simulink model "QCar2_CameraDriving"  (R2025b)
settings: Solver=ode2  StartTime=0.0  StopTime=inf  FixedStep=1/100  RelTol=1e-3  EnableMultiTasking=on
InitFcn:
  | modelFile = get_param(bdroot,'FileName');
  | modelDir  = fileparts(modelFile);
  | 
  | addpath(modelDir); % so load_waypoints.m is found if it sits next to the model
  | addpath(fullfile(modelDir,".."));
  | 
  | wpFile = fullfile(modelDir, "waypoints.txt");
  | WP = load_waypoints(wpFile);
  | 
  | assignin("base","WP",WP);
model workspace (MAT data in the model file):
  camera_rate : Simulink.Parameter (value not decoded)
  depth_rate : Simulink.Parameter (value not decoded)
symbols that are objects in the model workspace (value not decoded): camera_rate, depth_rate
undefined symbols (not defined in the file or in its folder): gcbh, HIL, JPEG, Point, qc_get_step_size, Video3D, video_display_show
libraries: quarc_library x37, simulink x14
(part 2 of 3)

== system QCar2_CameraDriving/monitorTiming 2 ==
  note: moniorTiming Module:
      |
      | This subsystem outputs the sample time and computation time of the model.
      |
      | Outputs:
      | sampleTime (s) n/a : Sample time (unfiltered and filtered) in seconds.
      | computationTime (s) n/a : Computation time (unfiltered and filtered) in seconds.
      |
      | Usage:
      | Compare the Sample Time (s) output to a constant (qc_get_step_size) to monitor whether or not the desired sample time is being achieved. The Computation Time (s) values should be lower than the corresponding sample time value to ensure that the solver has enough time per time step.
  note: Timing Performance
  Computation Time : quarc_library/Sources/Time/Computation Time  sample_time=depth_rate  use_model=on  use_cpu_time=off
  Constant : Constant  Value=depth_rate  SampleTime=depth_rate
  Mux : Mux  Inputs=2
  Sample Time : quarc_library/Sources/Time/Sample Time  Priority=-99  sample_time=depth_rate
  sampleTime (s) : Outport  VectorParamsAs1DForOutWhenUnconnected=off
  computationTime (s) : Outport  Port=2  VectorParamsAs1DForOutWhenUnconnected=off
  wires:
  Constant/1 -> Mux/2
  Sample Time/1 -> Mux/1
  Mux/1 -> sampleTime (s)/1
  Computation Time/1 -> computationTime (s)/1

== system QCar2_CameraDriving/monitorTiming 3 ==
  note: Timing Performance
  note: monitorTiming Module:
      |
      | This subsystem provides three timing signals for any given rate in your model.
      |
      | Outputs:
      | timing (s) n/a : Sample time, sample time reference and computation time in seconds.
      |
      | Usage:
      | Set the 'Sample time (seconds)' parameter in all three blocks below to the same number. This will provide the actual sample time at each time step, the reference sample time that is being targeted as well as the computation time of that particular loop in the model into one vector signal for scoping.
  Computation Time : quarc_library/Sources/Time/Computation Time  sample_time=qc_get_step_size  use_model=on  use_cpu_time=off
  Constant : Constant  Value=qc_get_step_size
  Mux : Mux  Inputs=3
  Sample Time : quarc_library/Sources/Time/Sample Time  Priority=-99  sample_time=qc_get_step_size
  timing (s) : Outport  VectorParamsAs1DForOutWhenUnconnected=off
  wires:
  Mux/1 -> timing (s)/1
  Computation Time/1 -> Mux/3  "computation time"
  Sample Time/1 -> Mux/1  "actual sample time"
  Constant/1 -> Mux/2  "reference"

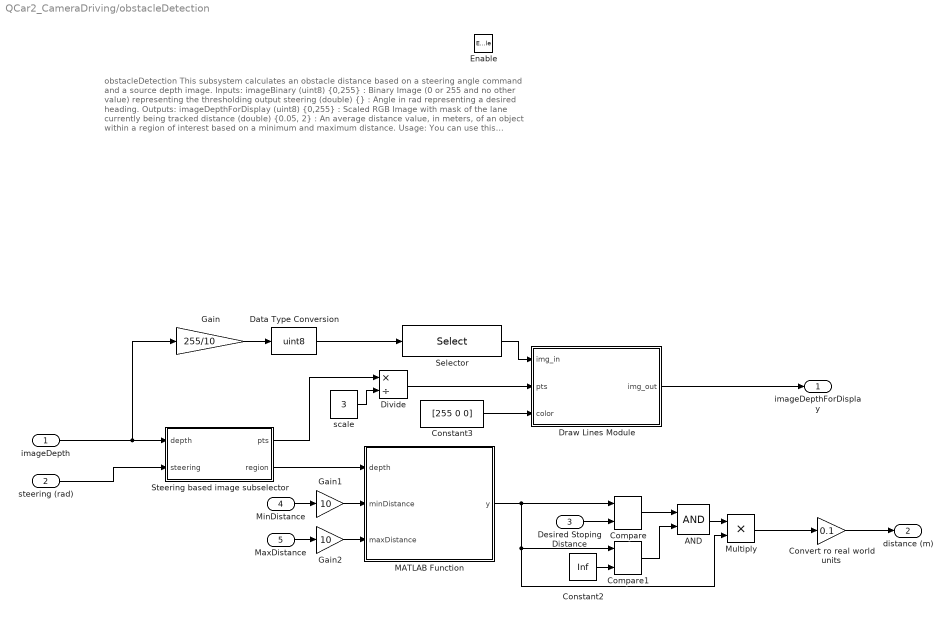
== system QCar2_CameraDriving/obstacleDetection ==
  note: obstacleDetection
      | This subsystem calculates an obstacle distance based on a steering angle command and a source depth image.
      |
      | Inputs:
      | imageBinary (uint8) {0,255} : Binary Image (0 or 255 and no other value) representing the thresholding output
      | steering (double) {} : Angle in rad representing a desired heading.
      |
      | Outputs:
      | imageDepthForDisplay (uint8) {0,255} : Scaled RGB Image with mask of the lane currently being tracked
      | distance (double) {0.05, 2} : An average distance value, in meters, of an object within a region of interest based on a minimum and maximum distance.
      |
      | Usage:
      |
      | You can use this subsystem to determine if the desired heading angle will cause the car to colllide with an obstacle by examining the distances from a region of interest within the depth image and calculating how far the obstacle is.
  imageDepth : Inport
  steering (rad) : Inport  Port=2
  Desired Stoping Distance : Inport  Port=3
  MinDistance : Inport  Port=4
  MaxDistance : Inport  Port=5
  Enable : EnablePort  PropagateVarSize=During execution
  AND : Logic  AllPortsSameDT=off  OutDataTypeStr=boolean
  Compare : quarc_library/Logic Operations/Compare  operator=>=  output_data_type=boolean
      settings: SourceProductName=QUARC Targets
  Compare1 : quarc_library/Logic Operations/Compare  operator=<  output_data_type=boolean
      settings: SourceProductName=QUARC Targets
  Constant2 : Constant  Value=Inf
  Constant3 : Constant  Value=[255 0 0]
  Convert ro real world units : Gain  Gain=0.1
  Data Type Conversion : DataTypeConversion  OutDataTypeStr=uint8  SaturateOnIntegerOverflow=off  RndMeth=Floor
  Divide : Product  Inputs=*/  OutDataTypeStr=Inherit: Inherit via back propagation
  Draw Lines Module : MATLAB Function  TreatAsAtomicUnit=on
  Gain : Gain  Gain=255/10
  Gain1 : Gain  Gain=10
  Gain2 : Gain  Gain=10
  MATLAB Function : MATLAB Function  TreatAsAtomicUnit=on
  Multiply : Product
  Selector : Selector  NumberOfDimensions=2  InputPortWidth=3  IndexOptions=Index vector (dialog),Index vector (dialog)  Indices=[1:3:360],[1:3:640]  OutputSizes=1,1
  Steering based image subselector : MATLAB Function  TreatAsAtomicUnit=on
  scale : Constant  Value=3
  imageDepthForDisplay : Outport  VectorParamsAs1DForOutWhenUnconnected=off
  distance (m) : Outport  Port=2  VectorParamsAs1DForOutWhenUnconnected=off
  wires:
  Constant3/1 -> Draw Lines Module/3(color)
  Steering based image subselector/1(pts) -> Divide/1
  Steering based image subselector/2(region) -> MATLAB Function/1(depth)
  steering (rad)/1 -> Steering based image subselector/2(steering)
  Multiply/1 -> Convert ro real world units/1
  MaxDistance/1 -> Gain2/1
  MinDistance/1 -> Gain1/1
  MATLAB Function/1(y) -> Compare/1, Multiply/2, Compare1/1
  imageDepth/1 -> Steering based image subselector/1(depth), Gain/1
  Selector/1 -> Draw Lines Module/1(img_in)
  Data Type Conversion/1 -> Selector/1
  Divide/1 -> Draw Lines Module/2(pts)
  Draw Lines Module/1(img_out) -> imageDepthForDisplay/1
  scale/1 -> Divide/2
  Gain/1 -> Data Type Conversion/1
  Desired Stoping Distance/1 -> Compare/2
  Compare/1 -> AND/1
  Compare1/1 -> AND/2
  Constant2/1 -> Compare1/2
  AND/1 -> Multiply/1
  Convert ro real world units/1 -> distance (m)/1
  Gain1/1 -> MATLAB Function/2(minDistance)
  Gain2/1 -> MATLAB Function/3(maxDistance)

== system QCar2_CameraDriving/odometry ==
  v_in : Inport
  steer_in : Inport  Port=2
  Ts_const : Constant  Value=0.02
  odometry_step : MATLAB Function  TreatAsAtomicUnit=on
  state_delay : UnitDelay  InitialCondition=[0;0;0]  SampleTime=-1  HasFrameUpgradeWarning=on
  pose_out : Outport
  wires:
  state_delay/1 -> odometry_step/1(prev_state)
  v_in/1 -> odometry_step/2(v)
  steer_in/1 -> odometry_step/3(steer)
  Ts_const/1 -> odometry_step/4(Ts)
  odometry_step/1(pose_next) -> state_delay/1, pose_out/1

== system QCar2_CameraDriving/pointCloud ==
  note: Convert LIDAR information to Point Cloud Image
  note: pointCloud Module:
      |
      | This subsystem generates a point cloud image based on LIDAR data.
      |
      | Inputs:
      | distances (m) n/a : Distances measured by LIDAR
      | headings (rad) n/a : Headings at which distances are measured
      |
      | Outputs:
      | map (px) {0, 1} : 400 x 400 point cloud image
      |
      | Usage:
      | The data is dynamically saturated based on the maximumDistance (m) constant. To prevent a circle with radius being the maximumDistance showing up in the point cloud as a result of this saturation, data points corresponding to this are dropped in the findXYContour function. The function contourToPointCloud updates pixels in the map to 1 at new locations, and decays older data at the rate specified by the decay parameter.
  distances (m) : Inport
  heading (rad) : Inport  Port=2
  Constant1 : Constant  Value=0
  Saturation Dynamic : simulink/Discontinuities/Saturation Dynamic  OutMin=[]  OutMax=[]  OutDataTypeStr=Inherit: Same as second input  OutDataType=fixdt(1, 16)  OutScaling=2^-10  DoSatur=off
  contourToPointCloud : MATLAB Function  TreatAsAtomicUnit=on
  decay : Constant  Value=0
  findXYContour : MATLAB Function  TreatAsAtomicUnit=on
  maximumDistance (m) : Constant  Value=4
  map : Outport  VectorParamsAs1DForOutWhenUnconnected=off
  wires:
  distances (m)/1 -> Saturation Dynamic/2
  contourToPointCloud/1(mapOut) -> map/1
  Saturation Dynamic/1 -> findXYContour/1(distances)
  maximumDistance (m)/1 -> findXYContour/3(d_max), Saturation Dynamic/1
  Constant1/1 -> Saturation Dynamic/3
  decay/1 -> contourToPointCloud/3(decay)
  findXYContour/1(X) -> contourToPointCloud/1(X)
  findXYContour/2(Y) -> contourToPointCloud/2(Y)
  heading (rad)/1 -> findXYContour/2(heading)

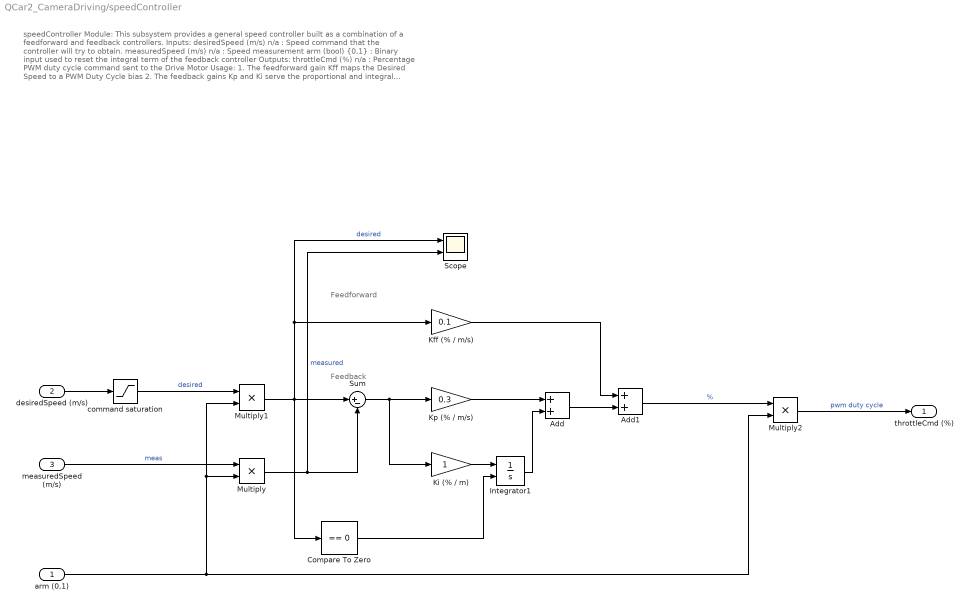
== system QCar2_CameraDriving/speedController ==
  note: Feedforward
  note: Feedback
  note: speedController Module:
      |
      | This subsystem provides a general speed controller built as a combination of a feedforward and feedback controllers.
      |
      | Inputs:
      | desiredSpeed (m/s) n/a : Speed command that the controller will try to obtain.
      | measuredSpeed (m/s) n/a : Speed measurement
      | arm (bool) {0,1} : Binary input used to reset the integral term of the feedback controller
      |
      | Outputs:
      | throttleCmd (%) n/a : Percentage PWM duty cycle command sent to the Drive Motor
      |
      | Usage:
      | 1. The feedforward gain Kff maps the Desired Speed to a PWM Duty Cycle bias
      | 2. The feedback gains Kp and Ki serve the proportional and integral terms to output corrections to the PWM Duty Cycle so as to regulate the desired speed.
  arm (0,1) : Inport
  desiredSpeed (m/s) : Inport  Port=2
  measuredSpeed (m/s) : Inport  Port=3
  Add : Sum
  Add1 : Sum
  Compare To Zero : simulink/Logic and Bit Operations/Compare To Zero  relop===  OutDataTypeStr=boolean
  Integrator1 : Integrator  ExternalReset=either  LimitOutput=on  UpperSaturationLimit=0.4  LowerSaturationLimit=-0.4
  Kff (% / m/s) : Gain  Gain=0.1
  "Ki (% / m) " : Gain
  Kp (% / m/s) : Gain  Gain=0.3
  Multiply : Product
  Multiply1 : Product
  Multiply2 : Product
  Scope : Scope  NumInputPorts=2
      settings: Title=Control Performance  ActiveDisplayYMinimum=0.76298814046961727  ActiveDisplayYMaximum=2.5122465814768962  YLabel=m/s
  Sum : Sum  Inputs=|+-
  command saturation : Saturate  UpperLimit=5  LowerLimit=-5
  throttleCmd (%) : Outport  VectorParamsAs1DForOutWhenUnconnected=off
  wires:
  command saturation/1 -> Multiply1/1  "desired"
  arm (0,1)/1 -> Multiply1/2, Multiply/2, Multiply2/2
  measuredSpeed (m/s)/1 -> Multiply/1  "meas"
  Multiply/1 -> Sum/2, Scope/2  "measured"
  Add/1 -> Add1/2
  Add1/1 -> Multiply2/1  "%"
  Multiply1/1 -> Compare To Zero/1, Sum/1, Kff (% / m/s)/1, Scope/1  "desired"
  Integrator1/1 -> Add/2
  Multiply2/1 -> throttleCmd (%)/1  "pwm duty cycle"
  Kp (% / m/s)/1 -> Add/1
  Compare To Zero/1 -> Integrator1/2
  Kff (% / m/s)/1 -> Add1/1
  Sum/1 -> "Ki (% / m) "/1, Kp (% / m/s)/1
  "Ki (% / m) "/1 -> Integrator1/1
  desiredSpeed (m/s)/1 -> command saturation/1

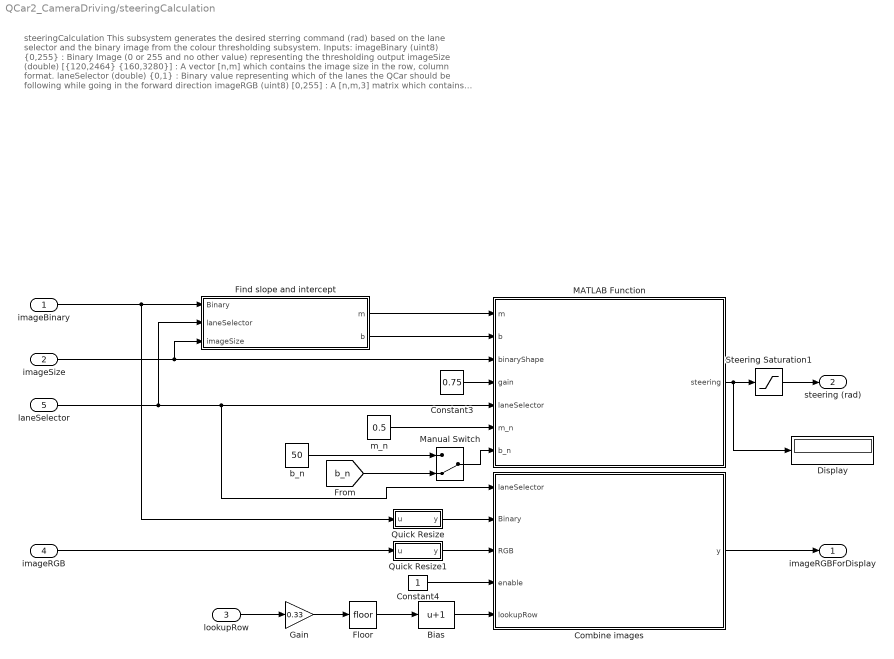
== system QCar2_CameraDriving/steeringCalculation ==
  note: steeringCalculation
      | This subsystem generates the desired sterring command (rad) based on the lane selector and the binary image from the colour thresholding subsystem.
      |
      | Inputs:
      | imageBinary (uint8) {0,255} : Binary Image (0 or 255 and no other value) representing the thresholding output
      | imageSize (double) [{120,2464} {160,3280}] : A vector [n,m] which contains the image size in the row, column format.
      | laneSelector (double) {0,1} : Binary value representing which of the lanes the QCar should be following while going in the forward direction
      | imageRGB (uint8) [0,255] : A [n,m,3] matrix which contains RGB values of an image in uint8 format
      |
      | Outputs:
      | steering (double) {-0.5,0.5} : Angle in rad representing the desired steering command based on the linearPolyFit
      | imageRGBForDisplay (uint8) {0,255} : A [n,m,3] matrix representing an RGB Image with mask of the lane currently being tracked
      |
      | Usage:
      |
      | This module can be used to generate a desired steering angle based on a thresheld image. A linear polygonal fit is used to generate a slope based on the equation y = mx+b whose slope and y intercept will define the steering angle commanded up to 0.5 (rad). The RGB image is a combination of the binary image holding information of the lane being followed, and a scaled version of the original RGB image.
  imageBinary : Inport
  imageSize : Inport  Port=2
  lookupRow : Inport  Port=3
  imageRGB : Inport  Port=4
  laneSelector : Inport  Port=5
  Bias : Bias  Bias=1  SaturateOnIntegerOverflow=off
  Combine images : MATLAB Function  TreatAsAtomicUnit=on
  Constant3 : Constant  Value=0.75
  Constant4 : Constant
  Display : Display
  Find slope and intercept : MATLAB Function  TreatAsAtomicUnit=on
  Floor : Rounding
  Gain : Gain  Gain=0.33
  MATLAB Function : MATLAB Function  TreatAsAtomicUnit=on
  Manual Switch : ManualSwitch  CurrentSetting=0
  Quick Resize : MATLAB Function  TreatAsAtomicUnit=on
  Quick Resize1 : MATLAB Function  TreatAsAtomicUnit=on
  Steering Saturation1 : Saturate
  b_n : Constant  Value=50
  m_n : Constant  Value=0.5
  imageRGBForDisplay : Outport  VectorParamsAs1DForOutWhenUnconnected=off
  steering (rad) : Outport  Port=2  VectorParamsAs1DForOutWhenUnconnected=off
  wires:
  Find slope and intercept/1(m) -> MATLAB Function/1(m)
  laneSelector/1 -> MATLAB Function/5(laneSelector), Combine images/1(laneSelector), Find slope and intercept/2(laneSelector)
  MATLAB Function/1(steering) -> Display/1, Steering Saturation1/1
  Constant3/1 -> MATLAB Function/4(gain)
  imageBinary/1 -> Quick Resize/1(u), Find slope and intercept/1(Binary)
  Find slope and intercept/2(b) -> MATLAB Function/2(b)
  Constant4/1 -> Combine images/4(enable)
  Quick Resize/1(y) -> Combine images/2(Binary)
  Quick Resize1/1(y) -> Combine images/3(RGB)
  Combine images/1(y) -> imageRGBForDisplay/1
  imageRGB/1 -> Quick Resize1/1(u)
  Steering Saturation1/1 -> steering (rad)/1
  Gain/1 -> Floor/1
  imageSize/1 -> Find slope and intercept/3(imageSize), MATLAB Function/3(binaryShape)
  lookupRow/1 -> Gain/1
  Bias/1 -> Combine images/5(lookupRow)
  Floor/1 -> Bias/1
  b_n/1 -> Manual Switch/1
  Manual Switch/1 -> MATLAB Function/7(b_n)
  [b_n] -> Manual Switch/2
  m_n/1 -> MATLAB Function/6(m_n)

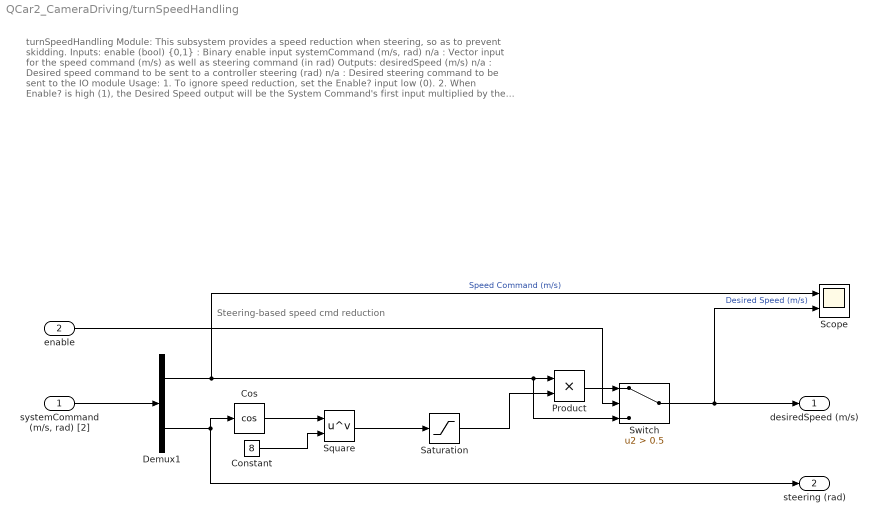
== system QCar2_CameraDriving/turnSpeedHandling ==
  note: turnSpeedHandling Module:
      |
      | This subsystem provides a speed reduction when steering, so as to prevent skidding.
      |
      | Inputs:
      | enable (bool) {0,1} : Binary enable input
      | systemCommand (m/s, rad) n/a : Vector input for the speed command (m/s) as well as steering command (in rad)
      |
      | Outputs:
      | desiredSpeed (m/s) n/a : Desired speed command to be sent to a controller
      | steering (rad) n/a : Desired steering command to be sent to the IO module
      |
      | Usage:
      | 1. To ignore speed reduction, set the Enable? input low (0).
      | 2. When Enable? is high (1), the Desired Speed output will be the System Command's first input multiplied by the cosine of the steering. Note that the lower limit of this reduction is set to 50% of the speed command input.
  note: Steering-based speed cmd reduction
  "systemCommand (m/s, rad) [2]" : Inport
  enable : Inport  Port=2
  Constant : Constant  Value=8
  Cos : Trigonometry  Operator=cos
  Demux1 : Demux  Outputs=2
  Product : Product
  Saturation : Saturate  UpperLimit=1  LowerLimit=0.5
  Scope : Scope  NumInputPorts=2
      settings: Title=Turn-Speed Handling  ActiveDisplayYMinimum=-2  ActiveDisplayYMaximum=2  YLabel=m/s  DataLoggingVariableName=ScopeData2
  Square : Math  Operator=pow  SignedPower=on
  Switch : Switch  Criteria=u2 > Threshold  Threshold=0.5  SaturateOnIntegerOverflow=off  InputSameDT=off
  desiredSpeed (m/s) : Outport  VectorParamsAs1DForOutWhenUnconnected=off
  steering (rad) : Outport  Port=2  VectorParamsAs1DForOutWhenUnconnected=off
  wires:
  Cos/1 -> Square/1
  Switch/1 -> desiredSpeed (m/s)/1, Scope/2  "Desired Speed (m/s)"
  Product/1 -> Switch/1
  Saturation/1 -> Product/2
  Demux1/1 -> Product/1, Switch/3, Scope/1  "Speed Command (m/s)"
  "systemCommand (m/s, rad) [2]"/1 -> Demux1/1
  enable/1 -> Switch/2
  Constant/1 -> Square/2
  Demux1/2 -> steering (rad)/1, Cos/1
  Square/1 -> Saturation/1

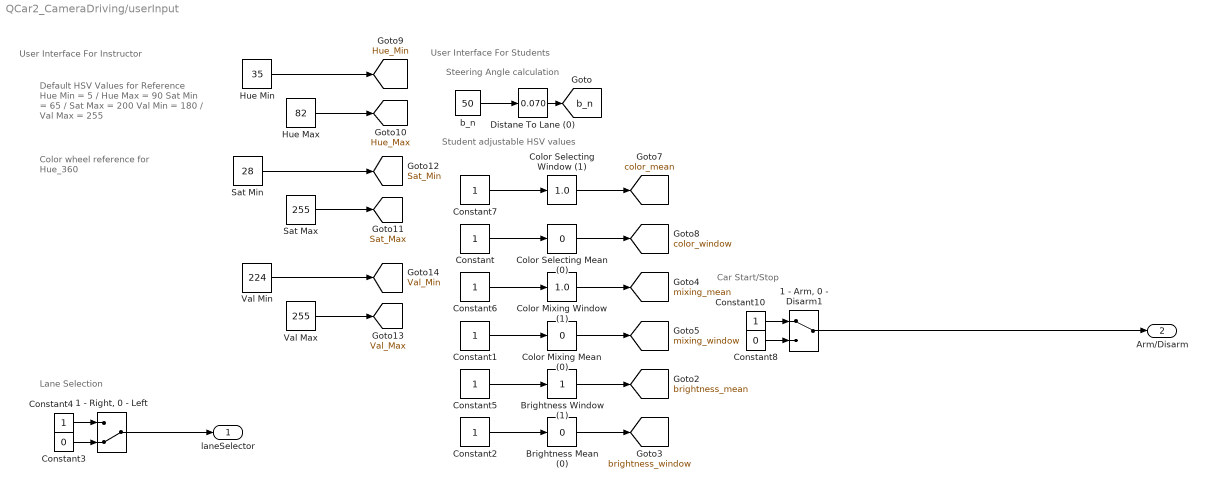
== system QCar2_CameraDriving/userInput ==
  note: Default HSV Values for Reference
      | Hue Min = 5 / Hue Max = 90
      | Sat Min = 65 / Sat Max = 200
      | Val Min = 180 / Val Max = 255
  note: User Interface For Instructor
  note: Student adjustable HSV values
  note: Lane Selection
  note: Car Start/Stop
  note: Steering Angle calculation
  note: User Interface For Students
  note: Color wheel
      | reference
      | for Hue_360
  "1 - Arm, 0 - Disarm1" : ManualSwitch
  "1 - Right, 0 - Left" : ManualSwitch  CurrentSetting=0
  Brightness Mean (0) : simulink/Math Operations/Slider Gain  gain=0  low=-1  high=1
  Brightness Window (1) : simulink/Math Operations/Slider Gain  gain=1  low=0  high=1
  Color Mixing Mean (0) : simulink/Math Operations/Slider Gain  gain=0  low=-1  high=1
  Color Mixing Window (1) : simulink/Math Operations/Slider Gain  gain=1.0  low=0  high=1
  Color Selecting Mean (0) : simulink/Math Operations/Slider Gain  gain=0  low=-1  high=1
  Color Selecting Window (1) : simulink/Math Operations/Slider Gain  gain=1.0  low=0  high=1
  Constant{,1..2,4..7,10} (8 alike) : Constant
  Constant3 : Constant  Value=0
  Constant8 : Constant  Value=0
  "Distane To Lane (0) " : simulink/Math Operations/Slider Gain  gain=0.070  low=0  high=1
  Hue Max : Constant  Value=82
  Hue Min : Constant  Value=35
  Sat Max : Constant  Value=255
  Sat Min : Constant  Value=28
  Val Max : Constant  Value=255
  Val Min : Constant  Value=224
  b_n : Constant  Value=50
  laneSelector : Outport  VectorParamsAs1DForOutWhenUnconnected=off
  Arm/Disarm : Outport  Port=2  VectorParamsAs1DForOutWhenUnconnected=off
  tag scope: Hue_Max=global, Hue_Min=global, Sat_Max=global, Sat_Min=global, Val_Max=global, Val_Min=global, b_n=global, brightness_mean=global, brightness_window=global, color_mean=global, color_window=global, mixing_mean=global, mixing_window=global
  wires:
  Constant3/1 -> "1 - Right, 0 - Left"/2
  "1 - Arm, 0 - Disarm1"/1 -> Arm/Disarm/1
  b_n/1 -> "Distane To Lane (0) "/1
  Constant4/1 -> "1 - Right, 0 - Left"/1
  Constant10/1 -> "1 - Arm, 0 - Disarm1"/1
  "1 - Right, 0 - Left"/1 -> laneSelector/1
  Constant8/1 -> "1 - Arm, 0 - Disarm1"/2
  "Distane To Lane (0) "/1 -> [b_n]
  Color Mixing Window (1)/1 -> [mixing_mean]
  Constant/1 -> Color Selecting Mean (0)/1
  Constant2/1 -> Brightness Mean (0)/1
  Constant5/1 -> Brightness Window (1)/1
  Constant1/1 -> Color Mixing Mean (0)/1
  Color Selecting Mean (0)/1 -> [color_window]
  Brightness Window (1)/1 -> [brightness_mean]
  Color Selecting Window (1)/1 -> [color_mean]
  Brightness Mean (0)/1 -> [brightness_window]
  Color Mixing Mean (0)/1 -> [mixing_window]
  Constant6/1 -> Color Mixing Window (1)/1
  Constant7/1 -> Color Selecting Window (1)/1
  Hue Min/1 -> [Hue_Min]
  Sat Min/1 -> [Sat_Min]
  Val Min/1 -> [Val_Min]
  Hue Max/1 -> [Hue_Max]
  Sat Max/1 -> [Sat_Max]
  Val Max/1 -> [Val_Max]

== system QCar2_CameraDriving/TrafficPerception_Python/TrafficTracking_Filter ==
  tl_state_raw : Inport  OutDataTypeStr=uint8
  stopSign_dist_raw : Inport  Port=2  OutDataTypeStr=double
  stop_required_raw : Inport  Port=3  OutDataTypeStr=boolean
  MATLAB Function : MATLAB Function  TreatAsAtomicUnit=on
  tl_stop : Outport  OutDataTypeStr=boolean
  sign_stop : Outport  Port=2  OutDataTypeStr=boolean
  stopSign_dist : Outport  Port=3  OutDataTypeStr=double
  wires:
  tl_state_raw/1 -> MATLAB Function/1(tl_state_raw)
  stopSign_dist_raw/1 -> MATLAB Function/3(stopSign_dist_raw)
  stop_required_raw/1 -> MATLAB Function/2(stop_required_raw)
  MATLAB Function/1(tl_stop) -> tl_stop/1
  MATLAB Function/2(sign_stop) -> sign_stop/1
  MATLAB Function/3(stopSign_dist) -> stopSign_dist/1

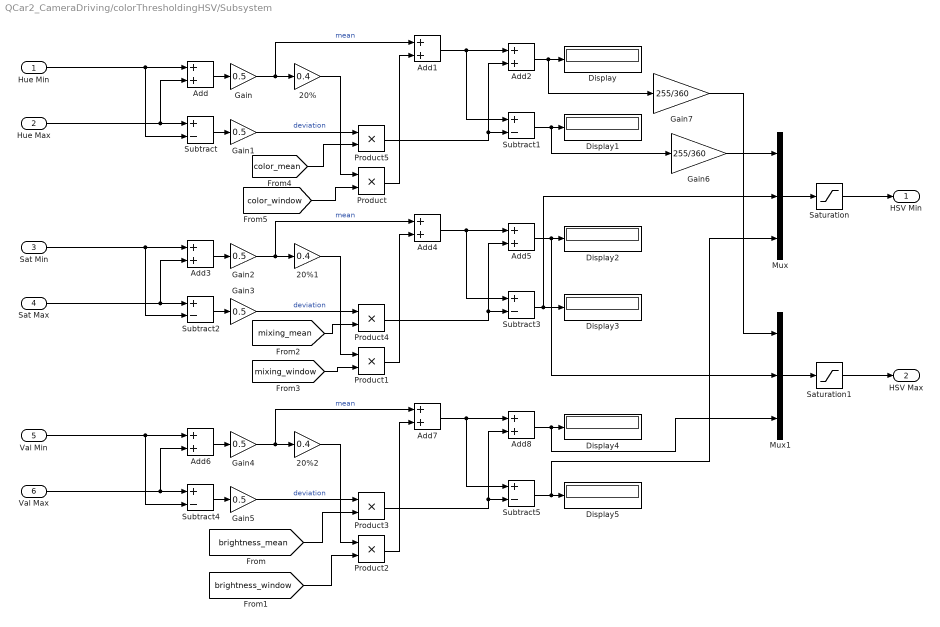
== system QCar2_CameraDriving/colorThresholdingHSV/Subsystem ==
  Hue Min : Inport
  Hue Max : Inport  Port=2
  Sat Min : Inport  Port=3
  Sat Max : Inport  Port=4
  Val Min : Inport  Port=5
  Val Max : Inport  Port=6
  20% : Gain  Gain=0.4
  20%1 : Gain  Gain=0.4
  20%2 : Gain  Gain=0.4
  Add{,1..8} (9 alike) : Sum
  Display{,1..5} (6 alike) : Display
  Gain{,1..5} (6 alike) : Gain  Gain=0.5
  Gain6 : Gain  Gain=255/360
  Gain7 : Gain  Gain=255/360
  Mux : Mux  Inputs=3
  Mux1 : Mux  Inputs=3
  Product{,1..5} (6 alike) : Product
  Saturation : Saturate  UpperLimit=[255 255 255]  LowerLimit=[0 0 0]
  Saturation1 : Saturate  UpperLimit=[255 255 255]  LowerLimit=[0 0 0]
  Subtract{,1..5} (6 alike) : Sum  Inputs=+-
  HSV Min : Outport  VectorParamsAs1DForOutWhenUnconnected=off
  HSV Max : Outport  Port=2  VectorParamsAs1DForOutWhenUnconnected=off
  wires:
  Product1/1 -> Add4/2
  Val Min/1 -> Add6/1, Subtract4/2
  Mux/1 -> Saturation/1
  Subtract1/1 -> Gain6/1, Display1/1
  Subtract4/1 -> Gain5/1
  Add1/1 -> Subtract1/1, Add2/1
  Product3/1 -> Add8/2, Subtract5/2
  Product2/1 -> Add7/2
  Gain4/1 -> 20%2/1, Add7/1  "mean"
  Add2/1 -> Gain7/1, Display/1
  Subtract3/1 -> Mux/2, Display3/1
  Subtract5/1 -> Mux/3, Display5/1
  Gain/1 -> 20%/1, Add1/1  "mean"
  Sat Min/1 -> Subtract2/2, Add3/1
  Subtract2/1 -> Gain3/1
  Product5/1 -> Add2/2, Subtract1/2
  Gain5/1 -> Product3/1  "deviation"
  Add5/1 -> Mux1/2, Display2/1
  Gain2/1 -> Add4/1, 20%1/1  "mean"
  Add8/1 -> Mux1/3, Display4/1
  Product/1 -> Add1/2
  Subtract/1 -> Gain1/1
  Product4/1 -> Subtract3/2, Add5/2
  Add4/1 -> Add5/1, Subtract3/1
  Add7/1 -> Subtract5/1, Add8/1
  Sat Max/1 -> Subtract2/1, Add3/2
  20%1/1 -> Product1/1
  [brightness_mean] -> Product3/2
  Mux1/1 -> Saturation1/1
  Add3/1 -> Gain2/1
  [mixing_mean] -> Product4/2
  Hue Min/1 -> Add/1, Subtract/2
  Hue Max/1 -> Add/2, Subtract/1
  Gain3/1 -> Product4/1  "deviation"
  Val Max/1 -> Add6/2, Subtract4/1
  20%2/1 -> Product2/1
  Add6/1 -> Gain4/1
  [color_window] -> Product/2
  [color_mean] -> Product5/2
  20%/1 -> Product/1
  Add/1 -> Gain/1
  Gain1/1 -> Product5/1  "deviation"
  [mixing_window] -> Product1/2
  [brightness_window] -> Product2/2
  Saturation/1 -> HSV Min/1
  Saturation1/1 -> HSV Max/1
  Gain6/1 -> Mux/1
  Gain7/1 -> Mux1/1

== matlab function QCar2_CameraDriving/steeringCalculation/Quick Resize1 ==
  data: u input; y output
function y = quickResize(u)

scale = 3;
    if length(size(u)) == 3
        y = u(1:scale:end, 1:scale:end, :);
    else
        y = u(1:scale:end, 1:scale:end);
    end

end

== matlab function QCar2_CameraDriving/automatedDriving/MATLAB Function ==
  data: obstacle_distance input; speed_cmd output; stop_distance input; nominal_tracking_distance input; nominal_speed input
function speed_cmd = adaptive_cruise_control(obstacle_distance, stop_distance, nominal_tracking_distance, nominal_speed)

speed_cmd = nominal_speed;

if obstacle_distance < stop_distance
    speed_cmd = 0;
    
elseif obstacle_distance < nominal_tracking_distance
    speed_cmd = nominal_speed/(nominal_tracking_distance-stop_distance)*obstacle_distance...
              - nominal_speed/(nominal_tracking_distance-stop_distance)*stop_distance;

end

== matlab function QCar2_CameraDriving/MATLAB Function ==
  data: imageRGB input; imageToThreshold output; laneSelector input; lookupRow input; imageSize output
function [imageToThreshold, imageSize]  = imageSelector(imageRGB, laneSelector, lookupRow)

[ROW, COL, ~] = size(imageRGB);
% imageToThreshold = uint8(zeros(ROW/2+1,COL/3,3));
if laneSelector
    imageToThreshold = imageRGB(round(ROW/2)+1:ROW, round(COL*(2/3)) + 1:COL, :);
else
    imageToThreshold = imageRGB(round(ROW/2)+1:ROW, 1:round(COL/3), :);
end
imageToThreshold(1: round(ROW/2) - (ROW - lookupRow + 1),:,:) = 0;
imageSize = [ROW - lookupRow + 1, round(COL/3)];

== matlab function QCar2_CameraDriving/TrafficPerception_Python/TrafficTracking_Filter/MATLAB Function ==
  data: tl_state_raw input; tl_stop output; stop_required_raw input; stopSign_dist_raw input; sign_stop output; stopSign_dist output
function [tl_stop, sign_stop, stopSign_dist] = trackFilter(tl_state_raw, stop_required_raw, stopSign_dist_raw)
% INPUT TYPES (enforce via Data Type Conversion blocks if needed):
%   tl_state_raw        : uint8  (0 unknown, 1 red, 2 yellow, 3 green)
%   stop_required_raw   : boolean
%   stopSign_dist_raw   : double (meters, Inf if none)
%
% OUTPUT TYPES:
%   tl_stop             : boolean
%   sign_stop           : boolean
%   stopSign_dist       : double
%
% Fixed sample time:
Ts = 1/30;  %#ok<NASGU>  % seconds (provided by you)

% ===== Tunables (in FRAMES, since Ts is fixed) =====
N_confirm = uint16(3);      % 3 frames @ 30 Hz = 0.1 s
T_hold_s  = 2.0;            % seconds
HOLD_STEPS = uint16(round(T_hold_s * 30));  % 2.0 * 30 = 60 frames

% ===== Persistent state =====
persistent redCount greenCount tlLatch
persistent signCount signLatch holdCount
persistent distHold

if isempty(redCount)
    redCount   = uint16(0);
    greenCount = uint16(0);
    tlLatch    = false;

    signCount  = uint16(0);
    signLatch  = false;
    holdCount  = uint16(0);

    distHold   = inf;
end

% ===== Helpers to prevent uint16 overflow wrapping =====
% (uint16 will wrap to 0 on overflow otherwise)
if redCount == intmax('uint16')
    redCount = intmax('uint16');
end
if greenCount == intmax('uint16')
    greenCount = intmax('uint16');
end
if signCount == intmax('uint16')
    signCount = intmax('uint16');
end

% ==============================
% A) TRAFFIC LIGHT: debounce + latch
% ==============================
isRed   = (tl_state_raw == uint8(1));
isGreen = (tl_state_raw == uint8(3));

% Count consecutive red frames
if isRed
    if redCount < intmax('uint16')
        redCount = redCount + 1;
    end
else
    redCount = uint16(0);
end

% Count consecutive green frames
if isGreen
    if greenCount < intmax('uint16')
        greenCount = greenCount + 1;
    end
else
    greenCount = uint16(0);
end

redConfirmed   = (redCount   >= N_confirm);
greenConfirmed = (greenCount >= N_confirm);

% Latch logic:
% - once red confirmed => tl_stop stays TRUE
% - only release after green confirmed => tl_stop becomes FALSE
if redConfirmed
    tlLatch = true;
elseif greenConfirmed
    tlLatch = false;
end

tl_stop = tlLatch;

% ==============================
% B) STOP SIGN: debounce + minimum hold timer
% ==============================
% Debounce
if stop_required_raw
    if signCount < intmax('uint16')
        signCount = signCount + 1;
    end
else
    signCount = uint16(0);
end

signConfirmed = (signCount >= N_confirm);

% Hold behavior:
% - when confirmed: latch TRUE and load holdCount = HOLD_STEPS
% - else: if holdCount>0 keep TRUE and decrement
% - else: FALSE
if signConfirmed
    signLatch = true;
    holdCount = HOLD_STEPS;
else
    if holdCount > 0
        holdCount = holdCount - 1;
        signLatch = true;
    else
        signLatch = false;
    end
end

sign_stop = signLatch;

% ==============================
% C) DISTANCE: hold last valid numeric measurement
% ==============================
% Keep last finite value in a sane range so Inf/NaN doesn't break downstream.
if isfinite(stopSign_dist_raw) && stopSign_dist_raw > 0.0 && stopSign_dist_raw < 1000.0
    distHold = stopSign_dist_raw;
end
stopSign_dist = distHold;

end

== stateflow chart QCar2_CameraDriving/MissionPlanner ==
  state TO_PICKUP
    entry:
    path_id = uint8(1);
    missionSpeed = V_CRUISE;
    missionStop = false;
    missionDone = false;
    pdCount = uint8(0);
    during:
    missionSpeed = V_CRUISE;
    missionStop = false;
    missionDone = false;
    if pathDone
    if pdCount < uint8(255)
    pdCount = pdCount + uint8(1);
    end
    else
    pdCount = uint8(0);
    end
  state DWELL_PICKUP
    entry:
    % Stop the car here (dwell)
    missionSpeed = 0.0;
    missionStop = true;
    missionDone = false;
    during:
    missionSpeed = 0.0;
    missionStop = true;
    missionDone = false;
  state TO_DROPOFF
    entry:
    path_id = uint8(2);
    missionSpeed = V_CRUISE;
    missionStop = false;
    missionDone = false;
    pdCount = uint8(0);
    during:
    missionSpeed = V_CRUISE;
    missionStop = false;
    missionDone = false;
    if pathDone
    if pdCount < uint8(255)
    pdCount = pdCount + uint8(1);
    end
    else
    pdCount = uint8(0);
    end
  state DWELL_DROPOFF
    entry:
    missionSpeed = 0.0;
    missionStop = true;
    missionDone = false;
    during:
    missionSpeed = 0.0;
    missionStop = true;
    missionDone = false;
  state TO_HUB
    entry:
    path_id = uint8(3);
    missionSpeed = V_CRUISE;
    missionStop = false;
    missionDone = false;
    pdCount = uint8(0);
    during:
    missionSpeed = V_CRUISE;
    missionStop = false;
    missionDone = false;
    if pathDone
    if pdCount < uint8(255)
    pdCount = pdCount + uint8(1);
    end
    else
    pdCount = uint8(0);
    end
  state DONE
    entry:
    missionSpeed = 0.0;
    missionStop = true;
    missionDone = true;
    during:
    missionSpeed = 0.0;
    missionStop = true;
    missionDone = true;
  (default) -> TO_PICKUP
  TO_HUB -> DONE : [pdCount >= uint8(3)]
  TO_PICKUP -> DWELL_PICKUP : [pdCount >= uint8(3)]
  DWELL_PICKUP -> TO_DROPOFF : [after(T_PICKUP, sec)]
  TO_DROPOFF -> DWELL_DROPOFF : [pdCount >= uint8(3)]
  DWELL_DROPOFF -> TO_HUB : [after(T_DROPOFF, sec)]
  data: pathDone input boolean size=1; path_id output uint8 size=1; missionSpeed output double; missionStop output boolean size=1; missionDone output boolean size=1; V_CRUISE constant double size=1 =3.0; T_PICKUP constant double size=1 =2.0; T_DROPOFF constant double size=1 =2.0; pdCount local uint8 =0

== matlab function QCar2_CameraDriving/pointCloud/contourToPointCloud ==
  data: X input size=720 [0..720]; mapOut output; Y input size=720; decay input
function mapOut = contourToPointCloud(X, Y, decay)
% Accumulate a 2D occupancy-like image from XY points (meters)
% X,Y can be vectors.

%#codegen

dim  = 400;   % image size dim x dim
gain = 50;    % pixels per meter

persistent mapInternal
if isempty(mapInternal)
    mapInternal = zeros(dim, dim);
else
    mapInternal = decay * mapInternal;
end

% Force column vectors
X = X(:);
Y = Y(:);

% 1-based center pixel
c = floor(dim/2) + 1;

% Map meters -> image coordinates
% col increases with +X, row decreases with +Y (typical image convention)
col = round(c + X * gain);
row = round(c - Y * gain);

% Keep only indices inside the image
valid = (row >= 1) & (row <= dim) & (col >= 1) & (col <= dim) ...
        & isfinite(row) & isfinite(col);

row = row(valid);
col = col(valid);

% If nothing valid, just output decayed map
if isempty(row)
    mapOut = mapInternal;
    return;
end

% Linear indexing (MATLAB is column-major): idx = row + (col-1)*dim
idx = row + (col - 1) * dim;

mapInternal(idx) = 1;
mapOut = mapInternal;
end

== matlab function QCar2_CameraDriving/WaypointTracker/wpTrack ==
  settings: updateMethod=DISCRETE
  data: W input; Nw input; pathDone output; x input; y input; yaw input; path_id input; psi_err output; wpIndex output uint16 size=[1 1]; distGoal output double size=[1 1]
function [pathDone, psi_err, wpIndex, distGoal] = wpTrack(W, Nw, x, y, yaw, path_id)
%#codegen
% W: 56x2 padded waypoints (double)
% Nw: uint16 true waypoint count (<=56)
% x,y,yaw: pose (double scalars)
% path_id: uint8 route selector
%
% psi_err OUTPUT IS NOW A "WAYPOINT STEERING COMMAND" (pure pursuit delta, radians)
% Positive delta = LEFT (matches what you told me)

% ---- vehicle params ----
L = 0.26;          % wheelbase (m) (match your odometry)
yaw_sign = 1.0;    % set to -1.0 ONLY if your yaw increases clockwise
delta_lim = 0.45;  % keep waypoint steering from overpowering lane keeping

persistent i lastPath doneLatch
if isempty(i),         i = uint16(1); end
if isempty(lastPath),  lastPath = uint8(255); end
if isempty(doneLatch), doneLatch = uint8(0); end

% Reset on path change
if path_id ~= lastPath
    i = uint16(1);
    lastPath = path_id;
    doneLatch = uint8(0);
end

% Guards
if ~isfinite(x) || ~isfinite(y) || ~isfinite(yaw)
    pathDone = false;
    psi_err  = 0.0;
    wpIndex  = i;
    distGoal = inf;
    return;
end

% Clamp N
N = uint16(Nw);
if N < uint16(1)
    pathDone = true;
    psi_err  = 0.0;
    wpIndex  = uint16(1);
    distGoal = 0.0;
    return;
end
if N > uint16(56)
    N = uint16(56);
end

% ---- tunables (path progress) ----
r_accept = 2.0;       % [m]
r_goal   = 3.0;       % [m]
r_accept2 = r_accept*r_accept;
r_goal2   = r_goal*r_goal;

% Ensure i in bounds
if i > N
    i = N;
end

% ---------------------------------------------------------------------
% 0) Find nearest waypoint (robust re-lock to path)
% Allow small backward correction (up to 5 points) if we drift
% ---------------------------------------------------------------------
nearestK = uint16(1);
bestD2 = inf;
for k = uint16(1):N
    kk = double(k);
    dxk = W(kk,1) - x;
    dyk = W(kk,2) - y;
    d2  = dxk*dxk + dyk*dyk;
    if d2 < bestD2
        bestD2 = d2;
        nearestK = k;
    end
end

if nearestK > i
    i = nearestK; % jump forward to nearest ahead
else
    % allow limited backward correction (prevents getting "stuck" off-path)
    if (i - nearestK) <= uint16(5)
        i = nearestK;
    end
end

% ---------------------------------------------------------------------
% 1) Advance waypoint index while close
% ---------------------------------------------------------------------
while i < N
    ii = double(i);
    dx = W(ii,1) - x;
    dy = W(ii,2) - y;
    if (dx*dx + dy*dy) < r_accept2
        i = i + uint16(1);
    else
        break;
    end
end

% ---------------------------------------------------------------------
% 2) Done detection + latch
% ---------------------------------------------------------------------
dxg = W(double(N),1) - x;
dyg = W(double(N),2) - y;
dGoal2 = dxg*dxg + dyg*dyg;

distGoal = sqrt(dGoal2);
doneNow  = (dGoal2 < r_goal2) || (i >= N);

if doneNow
    doneLatch = uint8(15); % latch for 15 ticks
else
    if doneLatch > uint8(0)
        doneLatch = doneLatch - uint8(1);
    end
end

pathDone = (doneLatch > uint8(0));
wpIndex  = i;

% ---------------------------------------------------------------------
% 3) Pure Pursuit waypoint steering (this is the "steering correction")
% Pick a target ahead by distance, not by fixed index (reduces corner cutting)
% ---------------------------------------------------------------------
Ld_des = 3.5;                % desired lookahead distance [m]
if distGoal < Ld_des
    Ld_des = max(1.5, distGoal); % shrink near end, but keep >=1.5m
end

% Find the first waypoint ahead of i whose distance >= Ld_des
j = i;
for k = i:N
    kk = double(k);
    dx = W(kk,1) - x;
    dy = W(kk,2) - y;
    d2 = dx*dx + dy*dy;
    if d2 >= (Ld_des*Ld_des)
        j = k;
        break;
    end
end

jj = double(j);
tx = W(jj,1);
ty = W(jj,2);

% Heading to target
yaw_eff = yaw_sign * yaw;
alpha = wrapToPi_local(atan2(ty - y, tx - x) - yaw_eff);

% Actual distance to target
dxT = tx - x;
dyT = ty - y;
Ld = sqrt(dxT*dxT + dyT*dyT);
if Ld < 1e-3
    psi_err = 0.0;
    return;
end

% Pure pursuit steering (delta), positive = left
delta = atan2(2.0*L*sin(alpha), Ld);

% Limit (prevents snapping into buildings when blended with lane steering)
if delta >  delta_lim
    delta =  delta_lim;
elseif delta < -delta_lim
    delta = -delta_lim;
end

psi_err = delta;   % keep name, but it's now a steering correction (rad)

end

function a = wrapToPi_local(a)
a = mod(a + pi, 2*pi) - pi;
end

== matlab function QCar2_CameraDriving/odometry/odometry_step ==
  data: prev_state input double size=[3 1]; pose_next output double size=[3 1]; v input double size=[1 1]; steer input double size=[1 1]; Ts input double size=[1 1]
function pose_next = odometry_step(prev_state, v, steer, Ts)
%#codegen
% prev_state: [x; y; yaw]  (3x1)
% v: m/s
% steer: rad
% Ts: sec

% Parameters
L = 0.26; % wheelbase (m)

x   = prev_state(1);
y   = prev_state(2);
yaw = prev_state(3);

% Kinematic bicycle model
x_dot   = v * cos(yaw);
y_dot   = v * sin(yaw);
yaw_dot = (v / L) * tan(steer);

% Euler integration
x_next   = x   + Ts * x_dot;
y_next   = y   + Ts * y_dot;
yaw_next = yaw + Ts * yaw_dot;

% wrap yaw to [-pi, pi]
yaw_next = atan2(sin(yaw_next), cos(yaw_next));

pose_next = [x_next; y_next; yaw_next];
end

== matlab function QCar2_CameraDriving/pointCloud/findXYContour ==
  data: distances input; X output size=720; heading input; Y output size=720; d_max input
function [X, Y] = findXYContour(distances, heading, d_max)

% find indices where distances corresponds to the d_max (bordering circle)
idx = distances < d_max;

% drop the bordering circle
temp_distances = distances(idx);
temp_heading = heading(idx);
% find X, Y pairs from distance, heading
X = temp_distances.*cos(temp_heading);
X_size = size(X);
Y = temp_distances.*sin(temp_heading);
Y_size = size(Y);

== matlab function QCar2_CameraDriving/LidarScanMatchICP ==
  data: lidar_pts input; pose output; dt input; isNew output
function [pose, isNew] = LidarScanMatchICP(lidar_pts, dt)
% Simulation-only LiDAR odometry using scan-to-scan ICP.
% pose = [x; y; yaw]

%#codegen
coder.extrinsic('icp_tform_4x4');

% --- Persistent numeric memory (NO empties)
persistent prevPts3 hasPrev T_global
if isempty(hasPrev)
    hasPrev  = false;
    prevPts3 = zeros(360,3);   % fixed-size
    T_global = eye(4);         % fixed-size
end

% --- Fixed-size outputs so Simulink can compile
pose = zeros(3,1);
isNew = false;

% Force expected shape (helps if Simulink treats as 1-D)
lidar_pts = reshape(lidar_pts, 360, 2);

% Build fixed 360x3 (z=0)
currPts3 = zeros(360,3);
currPts3(:,1:2) = lidar_pts;

% First scan initializes
if ~hasPrev
    prevPts3 = currPts3;
    hasPrev = true;
    isNew = true;
    return;
end

% Call extrinsic ICP helper: returns curr->prev
T = eye(4);  %#ok<NASGU>  % fixed-size for inference
T = icp_tform_4x4(currPts3, prevPts3);

% Integrate motion: prev->curr = inv(curr->prev)
T_inc = inv(T);
T_global = T_global * T_inc;

% Translation in rigid3d/affine3d matrix is in last row
x = T_global(4,1);
y = T_global(4,2);
yaw = atan2(T_global(2,1), T_global(1,1));

pose(:) = [x; y; yaw];
isNew = true;

% Update memory
prevPts3 = currPts3;
end

== matlab function QCar2_CameraDriving/EKF_Fuse ==
  settings: updateMethod=DISCRETE
  data: dt input; pose_out output; v_meas input; r_meas input; lidar_new input; lidar_pose input; ok output
function [pose_out, ok] = EKF_Fuse(dt, v_meas, r_meas, lidar_new, lidar_pose)
% EKF State: x = [X; Y; psi; v]
%#codegen

% ---- Force scalars (handles 1-D "vector with 1 element" signals)
dt        = double(dt(1));
v_meas    = double(v_meas(1));
r_meas    = double(r_meas(1));
lidar_new = logical(lidar_new(1));

% lidar_pose should be 3x1
lidar_pose = reshape(double(lidar_pose), 3, 1);

persistent x P initialized
if isempty(initialized)
    x = zeros(4,1); % [x;y;psi;v]
    P = diag([2^2, 2^2, (pi/2)^2, 1^2]);
    initialized = true;
end

% ---- Tunables
% IMPORTANT: use element-wise / scalar math (no matrix power)
q_xy  = (0.20*dt) * (0.20*dt);   % (m)^2 per step
q_psi = (0.03*dt) * (0.03*dt);   % (rad)^2 per step
q_v   = (0.80*dt) * (0.80*dt);   % (m/s)^2 per step
Q = diag([q_xy, q_xy, q_psi, q_v]);

R_v = 0.25 * 0.25;

% Avoid deg2rad() to keep it simple for codegen
sig_psi = 3*pi/180;
R_l = diag([0.10*0.10, 0.10*0.10, sig_psi*sig_psi]);

% ---- Predict
psi = x(3);
v   = x(4);

x_pred = x;
x_pred(1) = x(1) + v * dt * cos(psi);
x_pred(2) = x(2) + v * dt * sin(psi);
x_pred(3) = wrapToPi(x(3) + r_meas * dt);
% x_pred(4) stays v, corrected by wheel measurement

F = eye(4);
F(1,3) = -v * dt * sin(psi);
F(1,4) =  dt * cos(psi);
F(2,3) =  v * dt * cos(psi);
F(2,4) =  dt * sin(psi);

P = F*P*F.' + Q;

% ---- Update with wheel speed: z = v_meas
H_v = [0 0 0 1];
innov_v = v_meas - x_pred(4);
S = H_v*P*H_v.' + R_v;          % scalar
K = (P*H_v.') / S;              % 4x1
x_pred = x_pred + K*innov_v;
P = (eye(4) - K*H_v) * P;

% ---- Update with LiDAR pose: z = [x;y;psi]
if lidar_new
    H_l = [1 0 0 0;
           0 1 0 0;
           0 0 1 0];
    zhat  = x_pred(1:3);
    innov = lidar_pose - zhat;
    innov(3) = wrapToPi(innov(3));

    S = H_l*P*H_l.' + R_l;       % 3x3
    K = (P*H_l.') / S;           % 4x3
    x_pred = x_pred + K*innov;
    x_pred(3) = wrapToPi(x_pred(3));
    P = (eye(4) - K*H_l) * P;
end

x = x_pred;

pose_out = x(1:3);
ok = true;
end

function a = wrapToPi(x)
a = mod(x+pi, 2*pi) - pi;
end

== matlab function QCar2_CameraDriving/LidarPolarToCartesian ==
  data: dist input; pts output; ang input
function pts = LidarPolarToCartesian(dist, ang)
% Convert polar LiDAR scan to Cartesian point cloud (fixed size)
% dist, ang: 360x1 (or 1-D 360) -> output pts: 360x2

%#codegen

% Force column vectors (handles 1-D 360 too)
dist = dist(:);
ang  = ang(:);

N = numel(dist);      % should be 360

% Preallocate fixed-size output
pts = zeros(N,2);

% Compute all points (no size change)
pts(:,1) = dist .* cos(ang);
pts(:,2) = dist .* sin(ang);

% Invalidate bad ranges WITHOUT changing size
valid = (dist > 0.10) & (dist < 20.0) & isfinite(dist) & isfinite(ang);
pts(~valid,:) = NaN;     % (or 0) but NaN is easier to filter later
end

== matlab function QCar2_CameraDriving/obstacleDetection/Draw Lines Module ==
  data: img_in input; img_out output; pts input; color input
function img_out = drawLines(img_in, pts, color)

% Draw lines connecting the points using the provided color

% Inputs:
% img_in    : Input RGB Image (size = m by n)
% pts       : p x-y pairs of points (px) where markers are to be drawn
% color     : 1x3 matrix of RGB color values for each marker

% Outputs:
% img_out   : Output RGB Image with the markers drawn in (size = m by n)

%% Initialization
if size(img_in, 3) == 3
    img_out = img_in;
elseif size(img_in, 3) == 1
    img_out = cat(3, img_in, img_in, img_in);
end

[p, ~] = size(pts); % determine the number of points
%% Draw the lines
    for i = 1:p-1
        % determine the max(rows_difference, col_difference) between two
        % points
        itr = max(abs(pts(i,1) - pts(i+1,1)), abs(pts(i,2) - pts(i+1,2)));
        
        % generate linear spaces of row and col values between the pts
        row_vec = ceil(linspace(pts(i,1), pts(i+1,1), itr));
        col_vec = ceil(linspace(pts(i,2), pts(i+1,2), itr));
        
        % iterate through the values and shade them right

        for j = 1:itr
            img_out(row_vec(j), col_vec(j),1) = color(1);
            img_out(row_vec(j), col_vec(j),2) = color(2);
            img_out(row_vec(j), col_vec(j),3) = color(3);
        end
    end
end

== matlab function QCar2_CameraDriving/steeringCalculation/Find slope and intercept ==
  data: Binary input; m output; b output; laneSelector input; imageSize input
function [m, b] = linearPolyFit(Binary, laneSelector, imageSize)

% find the shape of the incoming image
[ROW, ~] = size(Binary);

% find row, col pairs of points where pixel value is bright
[rows, cols] = find(Binary(ROW - imageSize(1) + 1:end, :) > 0);

% x is coloumns, y is max_row - rows
if laneSelector
    x = imageSize(2) - cols;
else
    x = cols;
end

y = imageSize(1) - rows;

% fit a linear polynomial to the points and grab slope, intercept
% result = polyfit(x(idx), y(idx), 1);
result = polyfit(x, y, 1);
m = result(1); 
b = result(2);

== matlab function QCar2_CameraDriving/TrafficPerception_Python/pyDetect ==
  data: rgb input uint8 size=[410 820 3]; tl_state output uint8 size=[1 1]; depth input single size=[480 640]; stopDist output double size=[1 1]; stopRequired output boolean size=[1 1]
function [tl_state, stopDist, stopRequired] = pyDetect(rgb, depth)
% Sizes/types must be set in Ports & Data Manager:
%   rgb   : uint8 [<=Hmax <=Wmax 3]
%   depth : single/double [<=480 <=640]
% Outputs:
%   tl_state     : uint8 scalar
%   stopDist     : double scalar
%   stopRequired : boolean scalar

% Fixed typed defaults so Simulink can compile
tl_state = uint8(0);
stopDist = double(Inf);
stopRequired = false;

% Call a normal MATLAB function (NOT codegen) that does all Python work
coder.extrinsic('pyDetectWrapper');

[ts, sd, sr] = pyDetectWrapper(rgb, depth);

% Re-assert types (ts/sd/sr come back as mxArray)
tl_state = uint8(ts);
stopDist = double(sd);
stopRequired = logical(sr);
end

== matlab function QCar2_CameraDriving/steeringCalculation/MATLAB Function ==
  data: m input; steering output; b input; binaryShape input; gain input; laneSelector input; m_n input; b_n input
% function steering = fcn(m, b, binaryShape, gain, laneSelector, m_n, b_n)
% 
% % y = mx + b
% 
% current_x = (binaryShape(1) - b)/m;
% nominal_x = (binaryShape(1) - b_n)/m_n;
% if laneSelector
%     steering = -gain*(nominal_x - current_x)/binaryShape(2);
% else
%     steering = gain*(nominal_x - current_x)/binaryShape(2);
% end
function steering = fcn(m, b, binaryShape, gain, laneSelector, m_n, b_n)
%#codegen

% Hold last valid lane fit so steering never goes Inf
persistent m_hold b_hold
if isempty(m_hold)
    m_hold = m_n;
    b_hold = b_n;
end

% ---- validate binaryShape ----
if numel(binaryShape) < 2
    steering = 0.0;
    return;
end
y0 = double(binaryShape(1));
W  = double(binaryShape(2));
if ~isfinite(W) || W <= 1
    steering = 0.0;
    return;
end

% ---- validate m,b and fall back to held values ----
m_min = 1e-3;
if ~isfinite(m) || ~isfinite(b) || abs(m) < m_min
    m = m_hold;
    b = b_hold;
else
    m_hold = m;
    b_hold = b;
end

% ---- validate nominal params too ----
if ~isfinite(m_n) || abs(m_n) < m_min || ~isfinite(b_n)
    m_n = 0.5;
    b_n = 50;
end

% y = m x + b  ->  x = (y - b)/m
current_x = (y0 - b)  / m;
nominal_x = (y0 - b_n)/ m_n;

if ~isfinite(current_x) || ~isfinite(nominal_x)
    steering = 0.0;
    return;
end

e = (nominal_x - current_x) / W;

% laneSelector may be double/boolean; treat nonzero as true
if laneSelector ~= 0
    steering = -gain * e;
else
    steering =  gain * e;
end

% Clamp to match your Saturation block limits
if steering > 0.5
    steering = 0.5;
elseif steering < -0.5
    steering = -0.5;
end
end

== matlab function QCar2_CameraDriving/steeringCalculation/Quick Resize ==
  data: u input; y output
function y = quickResize(u)

scale = 3;
    if length(size(u)) == 3
        y = u(1:scale:end, 1:scale:end, :);
    else
        y = u(1:scale:end, 1:scale:end);
    end

end

== matlab function QCar2_CameraDriving/steeringCalculation/Combine images ==
  data: laneSelector input; Binary input; RGB input; y output size=[137,274,3]; enable input; lookupRow input
% function y = laneMask(laneSelector, Binary, RGB, enable, lookupRow)
% 
% y = RGB;
% [ROW, COL, ~] = size(y);
% [binRow, ~] = size(Binary);
% binarySection = Binary(binRow-(length(lookupRow:ROW))+1:binRow,:);
% if enable
%     if laneSelector
%         section = RGB(lookupRow:ROW, COL*(2/3) + 1:COL, :);
%         y(lookupRow:ROW, int16(COL*(2/3)) + 1:COL, 1) = ((255 - binarySection)/255).*section(:,:,1) + (binarySection).*section(:, :, 1);
%         y(lookupRow:ROW, int16(COL*(2/3)) + 1:COL, 2) = ((255 - binarySection)/255).*section(:,:,2);
%         y(lookupRow:ROW, int16(COL*(2/3)) + 1:COL, 3) = ((255 - binarySection)/255).*section(:,:,3);
%     else
%         section = RGB(lookupRow:ROW, 1:COL/3, :);
%         y(lookupRow:ROW, 1:int16(COL/3), 1) = ((255 - binarySection)/255).*section(:,:,1) + (binarySection).*section(:, :, 1);
%         y(lookupRow:ROW, 1:int16(COL/3), 2) = ((255 - binarySection)/255).*section(:,:,2);
%         y(lookupRow:ROW, 1:int16(COL/3), 3) = ((255 - binarySection)/255).*section(:,:,3);
%     end
% end
function y = laneMask(laneSelector, Binary, RGB, enable, lookupRow)
%#codegen

y = RGB;

if enable == 0
    return;
end

% Sizes
[ROWu, COLu, ~] = size(RGB);
[binRowu, binColu] = size(Binary);

ROW = int32(ROWu);
COL = int32(COLu);
binRow = int32(binRowu);
binCol = int32(binColu);

% ---- clamp lookupRow safely as int32 ----
lr = int32(floor(double(lookupRow)));  % force integer row
if lr < int32(1)
    lr = int32(1);
elseif lr > ROW
    lr = ROW;
end

% RGB row region
r1 = lr;
r2 = ROW;

roiH = r2 - r1 + int32(1);

% Clamp roiH to available Binary height; if clamped, shift r1 up
if roiH > binRow
    roiH = binRow;
    r1 = ROW - roiH + int32(1);
end

% Choose left or right third in RGB
if laneSelector ~= 0
    c1 = int32(floor(double(COL) * (2.0/3.0))) + int32(1);
    c2 = COL;
else
    c1 = int32(1);
    c2 = int32(floor(double(COL) * (1.0/3.0)));
end

% Ensure valid columns
if c1 < int32(1), c1 = int32(1); end
if c2 > COL,      c2 = COL;      end
if c2 < c1
    return;
end

regW = c2 - c1 + int32(1);

% Clamp overlay width to Binary width
useW = regW;
if useW > binCol
    useW = binCol;
    c2 = c1 + useW - int32(1);
end

% Binary bottom roiH rows
br1 = binRow - roiH + int32(1);
br2 = binRow;

binSec = Binary(br1:br2, 1:useW);

% Logical mask and uint8 versions
mask = (binSec ~= uint8(0));
m8  = uint8(mask);     % 0/1
nm8 = uint8(~mask);    % 0/1

% Extract RGB section
sec = y(r1:r2, c1:c2, :);

% Overlay red where mask is 1
sec(:,:,1) = nm8 .* sec(:,:,1) + m8 .* uint8(255);
sec(:,:,2) = nm8 .* sec(:,:,2);
sec(:,:,3) = nm8 .* sec(:,:,3);

% Write back
y(r1:r2, c1:c2, :) = sec;

end

== matlab function QCar2_CameraDriving/obstacleDetection/MATLAB Function ==
  data: depth input; y output; minDistance input; maxDistance input
function y = calculateDistance(depth, minDistance, maxDistance)

% This function drops depth data when outside the minDistance:maxDistance
% bounds and then averages the result. 

% u_flat = reshape(depth, 1, []);
% u_flat(u_flat < minDistance) = [];
% u_flat(u_flat > maxDistance) = [];
% y = mean(mean(u_flat));


u_flat = depth(depth <maxDistance);

u_flat  = depth(u_flat>minDistance);

y = mean(u_flat);
